simulink library "dyn_lib"  (R2023b)
settings: Solver=VariableStepAuto  StartTime=0.0  StopTime=10.0  RelTol=1e-3
undefined symbols (not defined in the file or in its folder): earth_radius, sun_radius, v0, x0
libraries: $bdroot x5, vrlib x3, matrix_library x1
settings Model: Creator=brent  LastModifiedBy=brent

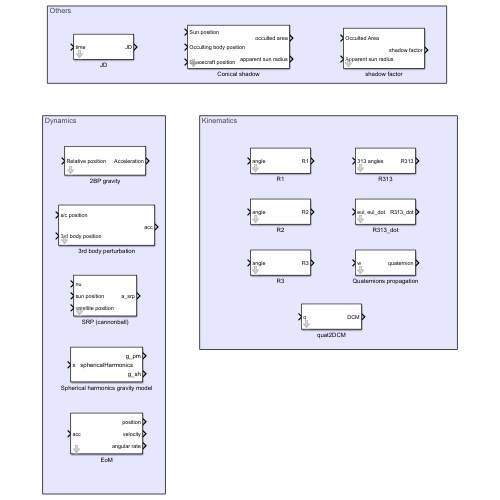
[thumbnail: Simulink's stored preview of the top-level diagram]
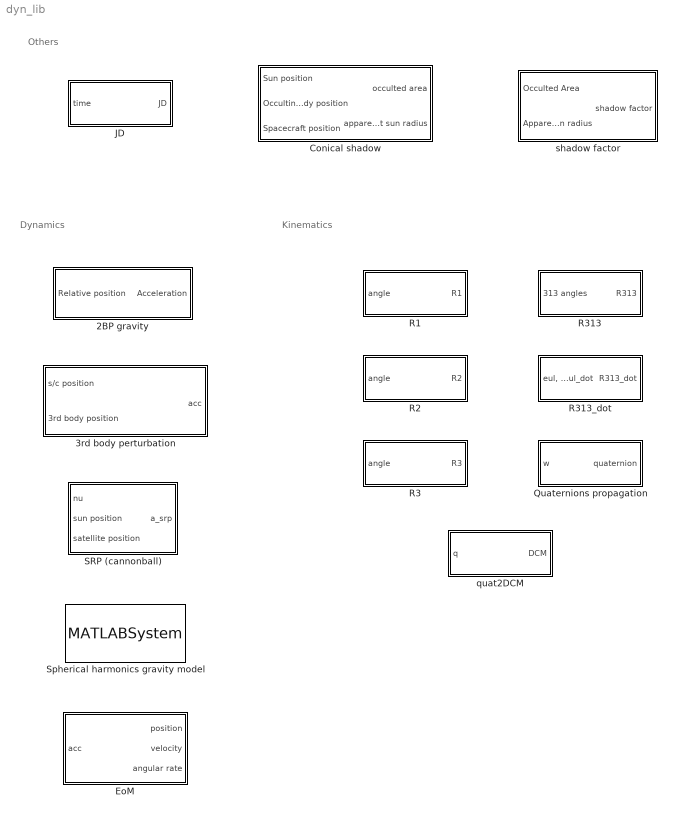
== system dyn_lib ==
  note: Kinematics
  note: Others
  note: Dynamics
  2BP gravity : Subsystem  mask{mu=0}
      mask prompts: mu "Celestial body's gravitational constant"
      mask DialogControl DescGroupVar Prompt: 2BP gravity
      mask DialogControl DescTextVar Prompt: Gravitational acceleration caused by one point mass, according to the two-body problem theory
  3rd body perturbation : Subsystem  mask{mu=sqrt(3)^3}
      mask prompts: mu "3rd body mu"
      mask DialogControl DescGroupVar Prompt: 3rd body perturbation
  Conical shadow : Subsystem  mask{R_B=earth_radius, R_S=sun_radius}
      mask prompts: R_B "Occulting body radius"; R_S "Sun Radius"
  EoM : Subsystem  mask{x0=x0, v0=v0}
      mask prompts: x0 "Initial position"; v0 "Initial velocity"
      mask DialogControl DescGroupVar Prompt: Equations of motion
  JD : Subsystem  mask{year=0, month=0, day=0, hour=0, min=0, sec=0}
      mask prompts: min "Minutes"; sec "Seconds"
      mask DialogControl DescGroupVar Prompt: Julian Date
      mask DialogControl DescTextVar Prompt: Compute the julian date computed as the sum of the parameter date and input seconds
      mask DialogControl ParameterGroupVar Prompt: Date
  Quaternions propagation : Subsystem  mask{q0=0}
      mask prompts: q0 "Initial attitude quaternion"
      mask DialogControl DescGroupVar Prompt: Quaternion propagation
  R1 : Subsystem
      mask DialogControl DescGroupVar Prompt: R1
      mask DialogControl DescTextVar Prompt: Rotate the reference frame of an angle alpha around the x axis. To rotate a vector and keep constant the reference frame, premultiply the vector by the transpose of this matrix
  R2 : Subsystem
      mask DialogControl DescGroupVar Prompt: R2
      mask DialogControl DescTextVar Prompt: Rotate the reference frame of an angle alpha around the y axis. To rotate a vector and keep constant the reference frame, premultiply the vector by the transpose of this matrix
  R3 : Subsystem
      mask DialogControl DescGroupVar Prompt: R3
      mask DialogControl DescTextVar Prompt: Rotate the reference frame of an angle alpha around the z axis. To rotate a vector and keep constant the reference frame, premultiply the vector by the transpose of this matrix.
  R313 : Subsystem
      mask DialogControl DescGroupVar Prompt: R313
      mask DialogControl DescTextVar Prompt: Rotate the reference frame with a 313 rotation series around the y axis. To rotate a vector and keep constant the reference frame, premultiply the vector by the transpose of this matrix
  R313_dot : Subsystem
      mask DialogControl DescGroupVar Prompt: R313_dot
      mask DialogControl DescTextVar Prompt: Time derivative of the 313 roation matrix
  SRP (cannonball) : Subsystem  mask{C_R=0, A_sc=0, m=0, AU=0, P=0}
      mask prompts: C_R "Radiation pressure coefficient"; A_sc "Spacecraft area"; m "Spacecraft mass"; AU "Astronomical units conversion"; P "Radiation pressure"
      mask DialogControl DescGroupVar Prompt: Solar Radiation Pressure
  Spherical harmonics gravity model : MATLABSystem  System=sphericalHarmonics  body_coeffs=[]  mu=[]  ref_radius=[]  nMax=[]  mMax=[]  SimulateUsing=Code generation
      mask Type: sphericalHarmonics
      mask Display:
      | disp('sphericalHarmonics');
      | port_label('input',1,'x');
      | port_label('output',1,'g_pm');
      | port_label('output',2,'g_sh');
  quat2DCM : Subsystem
      mask DialogControl DescGroupVar Prompt: quat2DCM
      mask DialogControl DescTextVar Prompt: convert a quaternion (scalar last) into the corresponding  rotation matrix
  shadow factor : Subsystem
      mask DialogControl DescGroupVar Prompt: Shadow factor

== system dyn_lib/2BP gravity ==
  note: $a = -\mu\frac{r}{|r|^3}$
  note: Two body problem equation
      |
      | Source:
      | H. D. Curtis, Orbital Mechanics for Engineering Students
  Relative position : Inport
  Constant : Constant  Value=3
  Constant1 : Constant  Value=mu
  Divide : Product  Inputs=*/
  Dot Product : DotProduct  OutDataTypeStr=Inherit: Inherit via internal rule
  Gain : Gain  Gain=-1
  Power : Math  Operator=pow
  Product : Product
  Square Root : Sqrt
  Acceleration : Outport
  wires:
  Square Root/1 -> Power/1
  Constant/1 -> Power/2
  Constant1/1 -> Divide/1
  Power/1 -> Divide/2
  Divide/1 -> Product/2
  Product/1 -> Gain/1
  Relative position/1 -> Dot Product/2, Dot Product/1, Product/1
  Dot Product/1 -> Square Root/1
  Gain/1 -> Acceleration/1

== system dyn_lib/3rd body perturbation ==
  note: $a = -\mu_3\frac{r_s - r_3}{|r_s - r_3|^3}$
  note: Gravitational perturbation due to the presence of a third body
      |
      | Source:
      | H. D. Curtis, Orbital Mechanics for Engineering Students
  s/c position : Inport
  3rd body position : Inport  Port=2
  2BP gravity : $bdroot/2BP gravity  mu=mu
  2BP gravity10 : $bdroot/2BP gravity  mu=mu
  Add2 : Sum  Inputs=+-
  Subtract : Sum
  acc : Outport
  wires:
  Add2/1 -> 2BP gravity/1
  s/c position/1 -> Add2/1  "satellite postion"
  2BP gravity/1 -> Subtract/1
  2BP gravity10/1 -> Subtract/2
  3rd body position/1 -> 2BP gravity10/1, Add2/2  "3rd body position"
  Subtract/1 -> acc/1  "acc"

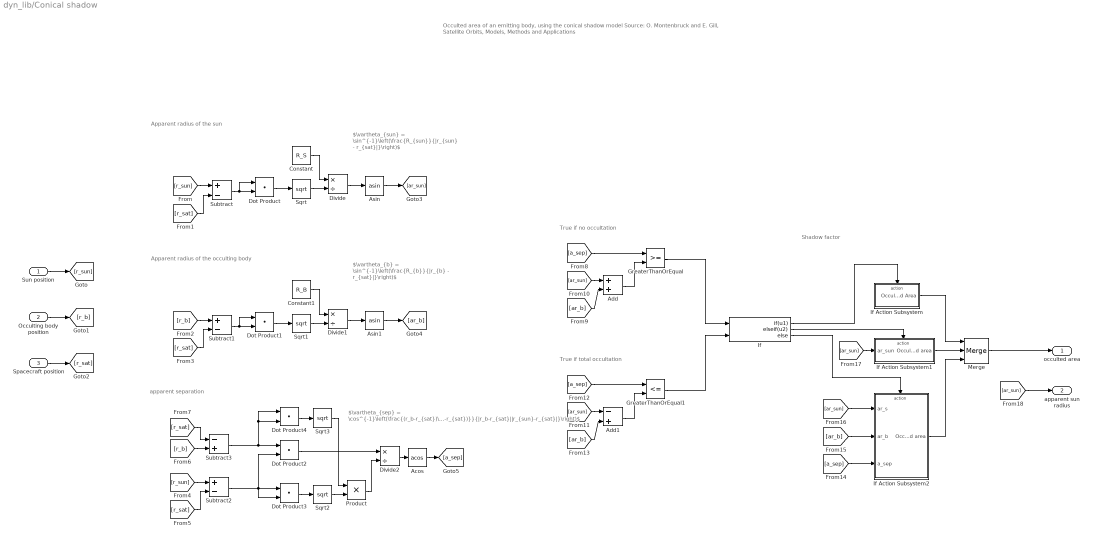
== system dyn_lib/Conical shadow ==
  note: $\vartheta_{b} = \sin^{-1}\left(\frac{R_{b}}{|r_{b} - r_{sat}|}\right)$
  note: Occulted area of an emitting body, using the conical shadow model
      |
      | Source:
      | O. Montenbruck and E. Gill, Satellite Orbits, Models, Methods and Applications
  note: Shadow factor
  note: True if no occultation
  note: apparent separation
  note: Apparent radius of the sun
  note: Apparent radius of the occulting body
  note: True if total occultation
  note: $\vartheta_{sun} = \sin^{-1}\left(\frac{R_{sun}}{|r_{sun} - r_{sat}|}\right)$
  note: $\vartheta_{sep} = \cos^{-1}\left(\frac{(r_b-r_{sat})\cdot{(r_{sun}-r_{sat})}}{|r_b-r_{sat}||r_{sun}-r_{sat}|}\right)$
  Sun position : Inport
  Occulting body position : Inport  Port=2
  Spacecraft position : Inport  Port=3
  Acos : Trigonometry  Operator=acos
  Add : Sum
  Add1 : Sum  Inputs=-+
  Asin : Trigonometry  Operator=asin
  Asin1 : Trigonometry  Operator=asin
  Constant : Constant  Value=R_S
  Constant1 : Constant  Value=R_B
  Divide : Product  Inputs=*/
  Divide1 : Product  Inputs=*/
  Divide2 : Product  Inputs=*/
  Dot Product{,1..4} (5 alike) : DotProduct  OutDataTypeStr=Inherit: Inherit via internal rule
  GreaterThanOrEqual : RelationalOperator  OutDataTypeStr=boolean  RndMeth=Simplest  InputSameDT=off
  GreaterThanOrEqual1 : RelationalOperator  Operator=<=  OutDataTypeStr=boolean  RndMeth=Simplest  InputSameDT=off
  If : If  NumInputs=2  IfExpression=u1  ElseIfExpressions=u2
  If Action Subsystem : Subsystem  TreatAsAtomicUnit=on
  If Action Subsystem1 : Subsystem  TreatAsAtomicUnit=on
  If Action Subsystem2 : Subsystem  TreatAsAtomicUnit=on
  Merge : Merge  Inputs=3
  Product : Product
  Sqrt{,1..3} (4 alike) : Sqrt
  Subtract : Sum  Inputs=+-
  Subtract1 : Sum  Inputs=+-
  Subtract2 : Sum  Inputs=+-
  Subtract3 : Sum  Inputs=-+
  occulted area : Outport
  apparent sun radius : Outport  Port=2
  wires:
  Divide2/1 -> Acos/1
  Acos/1 -> [a_sep]
  Sun position/1 -> [r_sun]
  Occulting body position/1 -> [r_b]
  Spacecraft position/1 -> [r_sat]
  [r_sun] -> Subtract/1
  [r_sat] -> Subtract/2
  Subtract/1 -> Dot Product/1, Dot Product/2
  Dot Product/1 -> Sqrt/1
  Constant/1 -> Divide/1
  Sqrt/1 -> Divide/2
  Divide/1 -> Asin/1
  Asin/1 -> [ar_sun]
  Asin1/1 -> [ar_b]
  Divide1/1 -> Asin1/1
  Sqrt1/1 -> Divide1/2
  Constant1/1 -> Divide1/1
  [r_b] -> Subtract1/1
  Dot Product1/1 -> Sqrt1/1
  Subtract1/1 -> Dot Product1/1, Dot Product1/2
  [r_sat] -> Subtract1/2
  [r_sun] -> Subtract2/1
  [r_sat] -> Subtract2/2
  [r_b] -> Subtract3/2
  [r_sat] -> Subtract3/1
  Subtract3/1 -> Dot Product4/2, Dot Product4/1, Dot Product2/1
  Subtract2/1 -> Dot Product3/2, Dot Product3/1, Dot Product2/2
  Dot Product2/1 -> Divide2/1
  Dot Product3/1 -> Sqrt2/1
  Dot Product4/1 -> Sqrt3/1
  Sqrt2/1 -> Product/2
  Sqrt3/1 -> Product/1
  Product/1 -> Divide2/2
  [a_sep] -> GreaterThanOrEqual/1
  [ar_sun] -> Add/1
  [ar_b] -> Add/2
  Add/1 -> GreaterThanOrEqual/2
  GreaterThanOrEqual/1 -> If/1
  If/1 -> If Action Subsystem/Action
  Add1/1 -> GreaterThanOrEqual1/2
  [a_sep] -> GreaterThanOrEqual1/1
  [ar_b] -> Add1/2
  GreaterThanOrEqual1/1 -> If/2
  [ar_sun] -> Add1/1
  If/2 -> If Action Subsystem1/Action
  If/3 -> If Action Subsystem2/Action
  [a_sep] -> If Action Subsystem2/3(a_sep)
  [ar_b] -> If Action Subsystem2/2(ar_b)
  [ar_sun] -> If Action Subsystem2/1(ar_s)
  If Action Subsystem1/1(Occulted area) -> Merge/2
  If Action Subsystem/1(Occulted Area) -> Merge/1
  If Action Subsystem2/1(Occulted area) -> Merge/3
  Merge/1 -> occulted area/1
  [ar_sun] -> If Action Subsystem1/1(ar_sun)
  [ar_sun] -> apparent sun radius/1

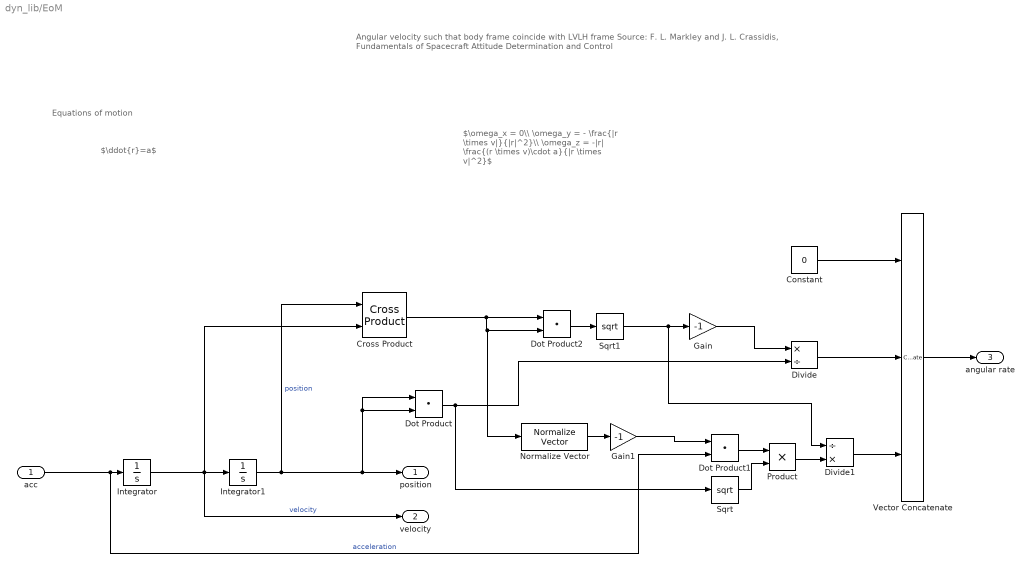
== system dyn_lib/EoM ==
  note: $\omega_x = 0\\ \omega_y = - \frac{|r \times v|}{|r|^2}\\ \omega_z = -|r| \frac{(r \times v)\cdot a}{|r \times v|^2}$
  note: Angular velocity such that body frame coincide with LVLH frame
      |
      | Source:
      | F. L. Markley and J. L. Crassidis, Fundamentals of Spacecraft Attitude Determination
      | and Control
  note: $\ddot{r}=a$
  note: Equations of motion
  acc : Inport
  Constant : Constant  Value=0
  Cross Product : matrix_library/Cross Product
  Divide : Product  Inputs=*/
  Divide1 : Product  Inputs=/*
  Dot Product : DotProduct  OutDataTypeStr=Inherit: Inherit via internal rule
  Dot Product1 : DotProduct  OutDataTypeStr=Inherit: Inherit via internal rule
  Dot Product2 : DotProduct  OutDataTypeStr=Inherit: Inherit via internal rule
  Gain : Gain  Gain=-1
  Gain1 : Gain  Gain=-1
  Integrator : Integrator  InitialCondition=v0
  Integrator1 : Integrator  InitialCondition=x0
  Normalize Vector : vrlib/Utilities/Normalize Vector  maxzero=0
  Product : Product
  Sqrt : Sqrt
  Sqrt1 : Sqrt
  Vector Concatenate : Concatenate  NumInputs=3
  position : Outport
  velocity : Outport  Port=2
  angular rate : Outport  Port=3
  wires:
  Normalize Vector/1 -> Gain1/1
  Gain/1 -> Divide/1
  Constant/1 -> Vector Concatenate/1
  Divide/1 -> Vector Concatenate/2
  Divide1/1 -> Vector Concatenate/3
  Sqrt1/1 -> Divide1/1, Gain/1
  Dot Product2/1 -> Sqrt1/1
  Product/1 -> Divide1/2
  Sqrt/1 -> Product/2
  Dot Product1/1 -> Product/1
  Gain1/1 -> Dot Product1/1
  Cross Product/1 -> Dot Product2/2, Normalize Vector/1, Dot Product2/1
  Dot Product/1 -> Sqrt/1, Divide/2
  Integrator/1 -> Cross Product/2, velocity/1, Integrator1/1  "velocity"
  acc/1 -> Dot Product1/2, Integrator/1  "acceleration"
  Integrator1/1 -> Cross Product/1, position/1, Dot Product/2, Dot Product/1  "position"
  Vector Concatenate/1 -> angular rate/1

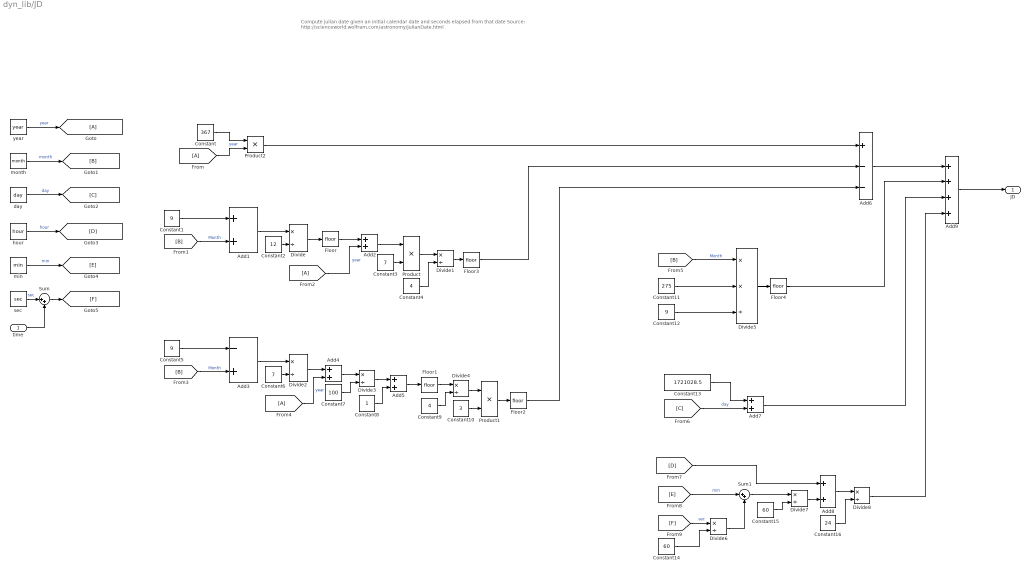
== system dyn_lib/JD ==
  note: Compute julian date given an initial calendar date and seconds elapsed from that date
      |
      | Source:
      | http://scienceworld.wolfram.com/astronomy/JulianDate.html
  time : Inport
  Add{1..2,4..5,7..8} (6 alike) : Sum
  Add3 : Sum  Inputs=-+
  Add6 : Sum  Inputs=+--
  Add9 : Sum  Inputs=++++
  Constant : Constant  Value=367
  Constant1 : Constant  Value=9
  Constant10 : Constant  Value=3
  Constant11 : Constant  Value=275
  Constant12 : Constant  Value=9
  Constant13 : Constant  Value=1721028.5
  Constant14 : Constant  Value=60
  Constant15 : Constant  Value=60
  Constant16 : Constant  Value=24
  Constant2 : Constant  Value=12
  Constant3 : Constant  Value=7
  Constant4 : Constant  Value=4
  Constant5 : Constant  Value=9
  Constant6 : Constant  Value=7
  Constant7 : Constant  Value=100
  Constant8 : Constant
  Constant9 : Constant  Value=4
  Divide{,1..4,6..8} (8 alike) : Product  Inputs=*/
  Divide5 : Product  Inputs=**/
  Floor{,1..4} (5 alike) : Rounding
  From : From
  From2 : From
  From4 : From
  Goto : Goto
  Product : Product
  Product1 : Product
  Product2 : Product
  Sum : Sum  Inputs=|++
  Sum1 : Sum  Inputs=|++
  day : Constant  Value=day
  hour : Constant  Value=hour
  min : Constant  Value=min
  month : Constant  Value=month
  sec : Constant  Value=sec
  year : Constant  Value=year
  JD : Outport
  wires:
  year/1 -> Goto/1  "year"
  month/1 -> [B]  "month"
  day/1 -> [C]  "day"
  Constant/1 -> Product2/1
  From/1 -> Product2/2  "year"
  [B] -> Add1/2  "Month"
  Constant1/1 -> Add1/1
  Add1/1 -> Divide/1
  Constant2/1 -> Divide/2
  Divide/1 -> Floor/1
  From2/1 -> Add2/2  "year"
  Floor/1 -> Add2/1
  Add2/1 -> Product/1
  Constant3/1 -> Product/2
  Product/1 -> Divide1/1
  Constant4/1 -> Divide1/2
  From4/1 -> Add4/2  "year"
  Add3/1 -> Divide2/1
  Constant7/1 -> Divide3/2
  Constant6/1 -> Divide2/2
  [B] -> Add3/2  "Month"
  Add4/1 -> Divide3/1
  Divide2/1 -> Add4/1
  Constant5/1 -> Add3/1
  Divide3/1 -> Add5/1
  Constant8/1 -> Add5/2
  Add5/1 -> Floor1/1
  Floor1/1 -> Divide4/1
  Constant9/1 -> Divide4/2
  Divide4/1 -> Product1/1
  Constant10/1 -> Product1/2
  Product1/1 -> Floor2/1
  Divide1/1 -> Floor3/1
  Product2/1 -> Add6/1
  Floor3/1 -> Add6/2
  Floor2/1 -> Add6/3
  [B] -> Divide5/1  "Month"
  Constant11/1 -> Divide5/2
  Constant12/1 -> Divide5/3
  [C] -> Add7/2  "day"
  Constant13/1 -> Add7/1
  min/1 -> [E]  "min"
  hour/1 -> [D]  "hour"
  sec/1 -> Sum/1  "sec"
  time/1 -> Sum/2
  Sum/1 -> [F]
  Constant14/1 -> Divide6/2
  [F] -> Divide6/1  "sec"
  Divide6/1 -> Sum1/2
  [E] -> Sum1/1  "min"
  Sum1/1 -> Divide7/1
  Constant15/1 -> Divide7/2
  Divide7/1 -> Add8/2
  [D] -> Add8/1
  Constant16/1 -> Divide8/2
  Add8/1 -> Divide8/1
  Add6/1 -> Add9/1
  Divide5/1 -> Floor4/1
  Add7/1 -> Add9/3
  Divide8/1 -> Add9/4
  Add9/1 -> JD/1
  Floor4/1 -> Add9/2

== system dyn_lib/Quaternions propagation ==
  note: $\dot{q} = \frac{1}{2}\Omega q$
  note: Quaternion propagation
      |
      | Source:
      | J. R. Wertz, Spacecraft Attitude Determination and Control
  w : Inport
  Create matrix OMEGA : Subsystem
  Gain : Gain  Gain=1/2  SaturateOnIntegerOverflow=on  OutDataTypeStr=Inherit: Same as input  ParamDataTypeStr=Inherit: Same as input
  Integrator2 : Integrator  InitialCondition=q0
  Matrix Multiply : Product  Multiplication=Matrix(*)
  Normalize Vector : vrlib/Utilities/Normalize Vector  maxzero=0
  quaternion : Outport
  wires:
  w/1 -> Create matrix OMEGA/1(w)
  Matrix Multiply/1 -> Integrator2/1  "q_dot"
  Normalize Vector/1 -> quaternion/1, Matrix Multiply/2  "q_norm"
  Integrator2/1 -> Normalize Vector/1  "q"
  Create matrix OMEGA/1(OMEGA) -> Gain/1
  Gain/1 -> Matrix Multiply/1

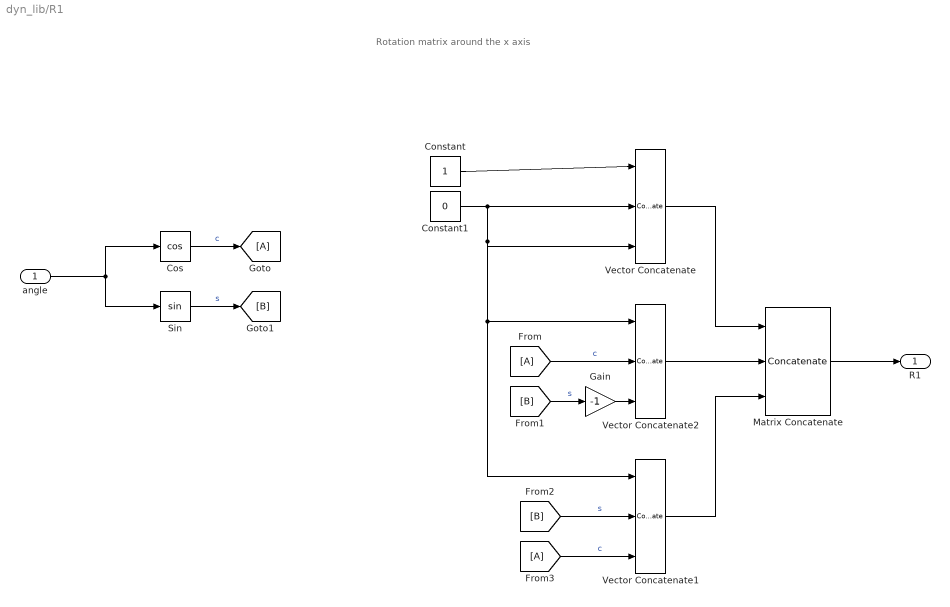
== system dyn_lib/R1 ==
  note: Rotation matrix around the x axis
  angle : Inport
  Constant : Constant
  Constant1 : Constant  Value=0
  Cos : Trigonometry  Operator=cos
  From : From
  From3 : From
  Gain : Gain  Gain=-1
  Goto : Goto
  Matrix Concatenate : Concatenate  NumInputs=3  Mode=Multidimensional array  ConcatenateDimension=2
  Sin : Trigonometry
  Vector Concatenate : Concatenate  NumInputs=3
  Vector Concatenate1 : Concatenate  NumInputs=3
  Vector Concatenate2 : Concatenate  NumInputs=3
  R1 : Outport
  wires:
  angle/1 -> Cos/1, Sin/1
  Cos/1 -> Goto/1  "c"
  Sin/1 -> [B]  "s"
  Constant/1 -> Vector Concatenate/1
  Constant1/1 -> Vector Concatenate/2, Vector Concatenate/3, Vector Concatenate1/1, Vector Concatenate2/1
  From/1 -> Vector Concatenate2/2  "c"
  [B] -> Gain/1  "s"
  Gain/1 -> Vector Concatenate2/3
  [B] -> Vector Concatenate1/2  "s"
  From3/1 -> Vector Concatenate1/3  "c"
  Vector Concatenate2/1 -> Matrix Concatenate/2
  Vector Concatenate1/1 -> Matrix Concatenate/3
  Vector Concatenate/1 -> Matrix Concatenate/1
  Matrix Concatenate/1 -> R1/1

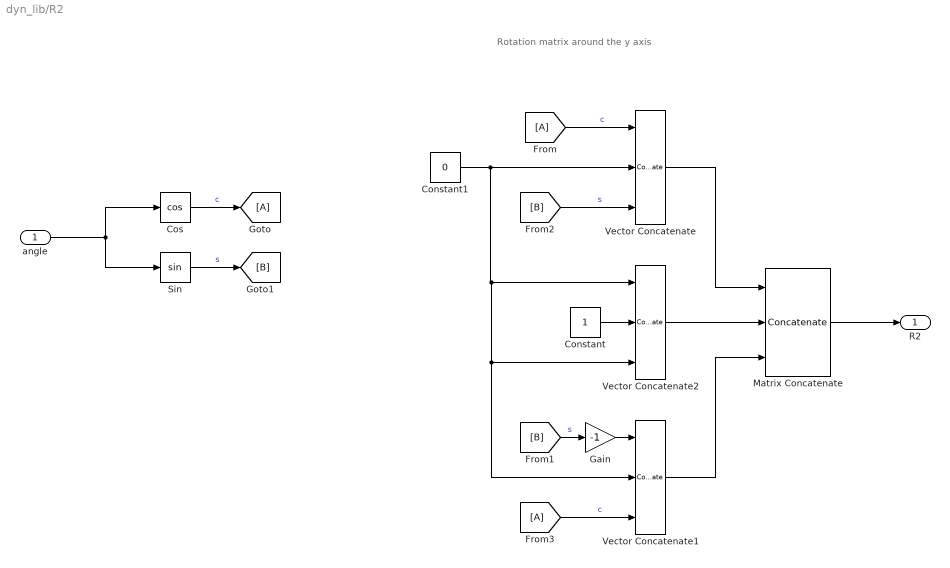
== system dyn_lib/R2 ==
  note: Rotation matrix around the y axis
  angle : Inport
  Constant : Constant
  Constant1 : Constant  Value=0
  Cos : Trigonometry  Operator=cos
  From : From
  From3 : From
  Gain : Gain  Gain=-1
  Goto : Goto
  Matrix Concatenate : Concatenate  NumInputs=3  Mode=Multidimensional array  ConcatenateDimension=2
  Sin : Trigonometry
  Vector Concatenate : Concatenate  NumInputs=3
  Vector Concatenate1 : Concatenate  NumInputs=3
  Vector Concatenate2 : Concatenate  NumInputs=3
  R2 : Outport
  wires:
  Matrix Concatenate/1 -> R2/1
  Vector Concatenate2/1 -> Matrix Concatenate/2
  Vector Concatenate/1 -> Matrix Concatenate/1
  Vector Concatenate1/1 -> Matrix Concatenate/3
  [B] -> Gain/1  "s"
  Cos/1 -> Goto/1  "c"
  Sin/1 -> [B]  "s"
  angle/1 -> Cos/1, Sin/1
  From/1 -> Vector Concatenate/1  "c"
  Constant1/1 -> Vector Concatenate1/2, Vector Concatenate2/3, Vector Concatenate2/1, Vector Concatenate/2
  [B] -> Vector Concatenate/3  "s"
  Constant/1 -> Vector Concatenate2/2
  Gain/1 -> Vector Concatenate1/1
  From3/1 -> Vector Concatenate1/3  "c"

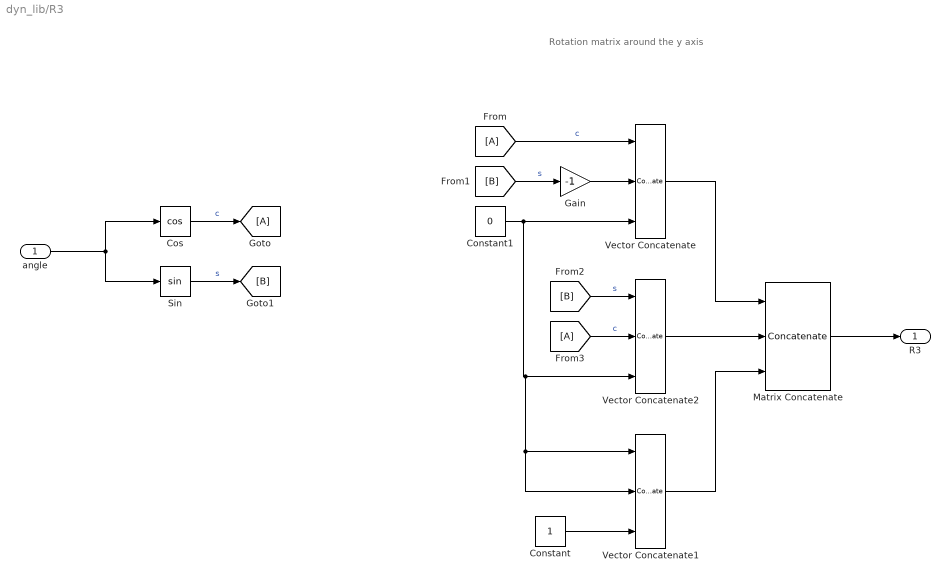
== system dyn_lib/R3 ==
  note: Rotation matrix around the y axis
  angle : Inport
  Constant : Constant
  Constant1 : Constant  Value=0
  Cos : Trigonometry  Operator=cos
  From : From
  From3 : From
  Gain : Gain  Gain=-1
  Goto : Goto
  Matrix Concatenate : Concatenate  NumInputs=3  Mode=Multidimensional array  ConcatenateDimension=2
  Sin : Trigonometry
  Vector Concatenate : Concatenate  NumInputs=3
  Vector Concatenate1 : Concatenate  NumInputs=3
  Vector Concatenate2 : Concatenate  NumInputs=3
  R3 : Outport
  wires:
  Cos/1 -> Goto/1  "c"
  angle/1 -> Cos/1, Sin/1
  Sin/1 -> [B]  "s"
  Vector Concatenate2/1 -> Matrix Concatenate/2
  Vector Concatenate1/1 -> Matrix Concatenate/3
  [B] -> Gain/1  "s"
  Vector Concatenate/1 -> Matrix Concatenate/1
  Matrix Concatenate/1 -> R3/1
  From/1 -> Vector Concatenate/1  "c"
  Gain/1 -> Vector Concatenate/2
  Constant1/1 -> Vector Concatenate1/1, Vector Concatenate1/2, Vector Concatenate2/3, Vector Concatenate/3
  [B] -> Vector Concatenate2/1  "s"
  From3/1 -> Vector Concatenate2/2  "c"
  Constant/1 -> Vector Concatenate1/3

== system dyn_lib/R313 ==
  note: Rotation matrix for the ZXZ sequence of rotations
  313 angles : Inport
  Demux : Demux  Outputs=3
  Matrix Multiply : Product  Inputs=3  Multiplication=Matrix(*)
  R1 : $bdroot/R1
  R3_1 : $bdroot/R3
  R3_2 : $bdroot/R3
  R313 : Outport
  wires:
  313 angles/1 -> Demux/1
  Demux/1 -> R3_1/1
  Demux/2 -> R1/1
  Demux/3 -> R3_2/1
  Matrix Multiply/1 -> R313/1
  R1/1 -> Matrix Multiply/2
  R3_1/1 -> Matrix Multiply/1
  R3_2/1 -> Matrix Multiply/3

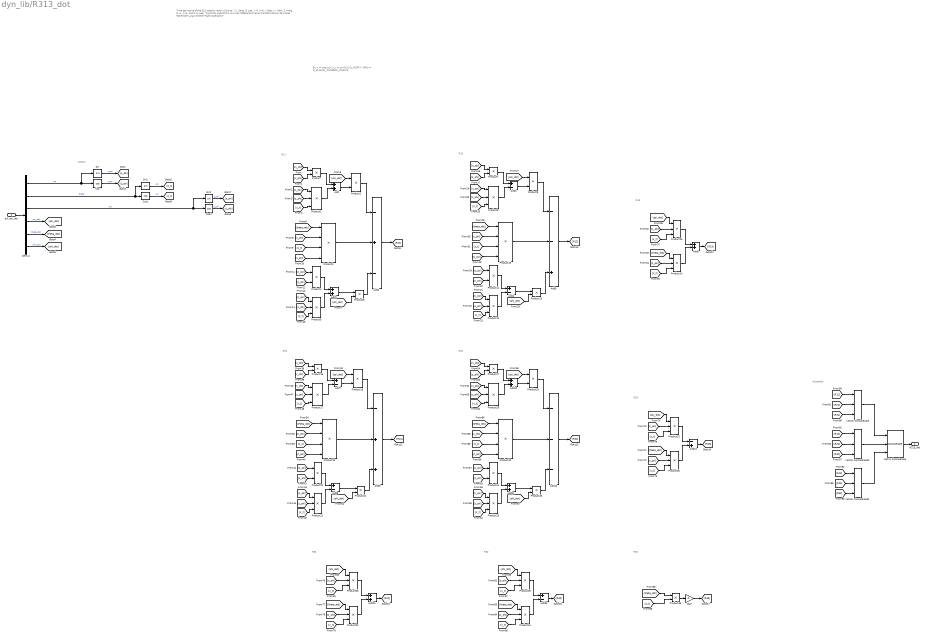
== system dyn_lib/R313_dot ==
  note: $c_x = \cos{x}\\ s_x = \sin{x}\\ D_{ICRF}^{PA} = R_3(\psi)R_1(\theta)R_3(\phi)$
  note: Time derivative of the 313 rotation matrix
      |
      | Source:
      | Y.-J. Song, D. Lee, Y.-R. Kim, J. Bae, J.-i. Park, S. Hong, D.-K. Kim, and S.-R. Lee, “Practical Algorithms on Lunar Reference Frame Transformations for Korea Pathfinder Lunar Orbiter Flight Operation”
  note: Assembly
  note: R13
  note: R11
  note: cos/sin
  note: R12
  note: R21
  note: R22
  note: R23
  note: R31
  note: R32
  note: R33
  "eul, eul_dot" : Inport
  Add{,1,6,10..11,14} (6 alike) : Sum
  Add12 : Sum  Inputs=---
  Add13 : Sum  Inputs=-+
  Add{3..4,7..8,15} (5 alike) : Sum  Inputs=+-
  Add2 : Sum  Inputs=-+-
  Add5 : Sum  Inputs=--+
  Add9 : Sum  Inputs=-++
  Cos : Trigonometry  Operator=cos
  Cos1 : Trigonometry  Operator=cos
  Cos2 : Trigonometry  Operator=cos
  Demux : Demux  Outputs=6
  Gain : Gain  Gain=-1
  Matrix Concatenate : Concatenate  NumInputs=3  Mode=Multidimensional array  ConcatenateDimension=2
  Product{,2,4,6..7,9,11,13,16,18,20,22,24,26..27,29,36} (17 alike) : Product
  Product{1,5,8,12,14..15,17,21,25,28,30..35} (16 alike) : Product  Inputs=3
  Product{3,10,19,23} (4 alike) : Product  Inputs=4
  Sin : Trigonometry
  Sin1 : Trigonometry
  Sin2 : Trigonometry
  Vector Concatenate : Concatenate  NumInputs=3
  Vector Concatenate1 : Concatenate  NumInputs=3
  Vector Concatenate2 : Concatenate  NumInputs=3
  R313_dot : Outport
  wires:
  "eul, eul_dot"/1 -> Demux/1
  Demux/1 -> Sin/1, Cos/1  "psi"
  Demux/4 -> [psi_dot]  "psi_dot"
  Demux/5 -> [theta_dot]  "theta_dot"
  Demux/6 -> [phi_dot]  "phi_dot"
  Demux/2 -> Sin1/1, Cos1/1  "theta"
  Demux/3 -> Cos2/1, Sin2/1  "phi"
  Sin/1 -> [s_psi]  "s_psi"
  Cos/1 -> [c_psi]  "c_psi"
  Sin1/1 -> [s_t]  "s_t"
  Cos1/1 -> [c_t]  "c_t"
  Sin2/1 -> [s_phi]  "s_phi"
  Cos2/1 -> [c_phi]  "c_phi"
  [s_psi] -> Product/1
  [c_phi] -> Product/2
  [s_phi] -> Product1/2
  [c_psi] -> Product1/1
  [c_t] -> Product1/3
  Product1/1 -> Add/2
  Product/1 -> Add/1
  Add/1 -> Product2/2
  [psi_dot] -> Product2/1
  [s_phi] -> Product3/2
  [s_t] -> Product3/3
  [theta_dot] -> Product3/1
  [s_psi] -> Product3/4
  [c_psi] -> Product4/1
  [s_phi] -> Product4/2
  [c_phi] -> Product5/2
  [c_t] -> Product5/3
  [s_psi] -> Product5/1
  Product5/1 -> Add1/2
  Product4/1 -> Add1/1
  Add1/1 -> Product6/1
  [phi_dot] -> Product6/2
  Product6/1 -> Add2/3
  Product3/1 -> Add2/2
  Product2/1 -> Add2/1
  Add2/1 -> [R11]
  [c_t] -> Product12/3
  [s_psi] -> Product10/4
  Product10/1 -> Add5/2
  [c_psi] -> Product11/1
  [theta_dot] -> Product10/1
  [c_phi] -> Product8/2
  Product9/1 -> Add5/1
  Product13/1 -> Add5/3
  [s_psi] -> Product12/1
  [s_psi] -> Product7/1
  [phi_dot] -> Product13/2
  [c_phi] -> Product10/2
  Add3/1 -> Product9/2
  [psi_dot] -> Product9/1
  [c_phi] -> Product11/2
  Product11/1 -> Add4/1
  [s_phi] -> Product7/2
  Product12/1 -> Add4/2
  [c_psi] -> Product8/1
  Product7/1 -> Add3/1
  Add4/1 -> Product13/1
  Product8/1 -> Add3/2
  [c_t] -> Product8/3
  Add5/1 -> [R12]
  [s_phi] -> Product12/2
  [s_t] -> Product10/3
  [s_psi] -> Product14/2
  [theta_dot] -> Product14/1
  [c_t] -> Product14/3
  [c_psi] -> Product15/2
  [psi_dot] -> Product15/1
  [s_t] -> Product15/3
  Product15/1 -> Add6/1
  Product14/1 -> Add6/2
  Add6/1 -> [R13]
  Add9/1 -> [R21]
  Product18/1 -> Add9/1
  Product19/1 -> Add9/2
  Product22/1 -> Add9/3
  [phi_dot] -> Product22/2
  Add8/1 -> Product22/1
  Product20/1 -> Add8/1
  Product21/1 -> Add8/2
  [c_psi] -> Product21/1
  [c_t] -> Product21/3
  [c_phi] -> Product21/2
  [s_phi] -> Product20/2
  [s_psi] -> Product20/1
  [c_psi] -> Product19/4
  [theta_dot] -> Product19/1
  [s_t] -> Product19/3
  [s_phi] -> Product19/2
  [psi_dot] -> Product18/1
  Add7/1 -> Product18/2
  Product16/1 -> Add7/1
  Product17/1 -> Add7/2
  [c_t] -> Product17/3
  [s_phi] -> Product17/1
  [s_psi] -> Product17/2
  [c_phi] -> Product16/2
  [c_psi] -> Product16/1
  Add11/1 -> Product26/1
  [s_phi] -> Product25/2
  [s_psi] -> Product28/1
  Product28/1 -> Add10/2
  Product27/1 -> Add10/1
  Product25/1 -> Add11/2
  Add12/1 -> [R22]
  [c_t] -> Product28/3
  [s_phi] -> Product27/2
  [c_psi] -> Product25/1
  [psi_dot] -> Product29/1
  Add10/1 -> Product29/2
  Product26/1 -> Add12/3
  [c_phi] -> Product24/2
  [c_psi] -> Product27/1
  Product24/1 -> Add11/1
  [c_phi] -> Product28/2
  Product29/1 -> Add12/1
  [phi_dot] -> Product26/2
  [s_psi] -> Product24/1
  [c_psi] -> Product23/4
  [s_t] -> Product23/3
  [theta_dot] -> Product23/1
  [c_t] -> Product25/3
  [c_phi] -> Product23/2
  Product23/1 -> Add12/2
  [c_t] -> Product30/3
  [psi_dot] -> Product31/1
  Product30/1 -> Add13/2
  [c_psi] -> Product30/2
  Product31/1 -> Add13/1
  [theta_dot] -> Product30/1
  Add13/1 -> [R23]
  [s_psi] -> Product31/2
  [s_t] -> Product31/3
  [theta_dot] -> Product32/1
  [s_t] -> Product33/3
  [c_phi] -> Product33/2
  [phi_dot] -> Product33/1
  [c_t] -> Product32/3
  Product33/1 -> Add14/1
  [s_phi] -> Product32/2
  Add14/1 -> [R31]
  Product32/1 -> Add14/2
  Product34/1 -> Add15/2
  [s_t] -> Product35/3
  [theta_dot] -> Product34/1
  [c_t] -> Product34/3
  [s_phi] -> Product35/2
  [phi_dot] -> Product35/1
  Add15/1 -> [R32]
  Product35/1 -> Add15/1
  [c_phi] -> Product34/2
  [theta_dot] -> Product36/1
  [s_t] -> Product36/2
  Product36/1 -> Gain/1
  Gain/1 -> [R33]
  Vector Concatenate2/1 -> Matrix Concatenate/2
  Vector Concatenate/1 -> Matrix Concatenate/1
  Vector Concatenate1/1 -> Matrix Concatenate/3
  [R11] -> Vector Concatenate/1
  [R21] -> Vector Concatenate/2
  [R31] -> Vector Concatenate/3
  [R22] -> Vector Concatenate2/2
  [R12] -> Vector Concatenate2/1
  [R32] -> Vector Concatenate2/3
  [R13] -> Vector Concatenate1/1
  [R23] -> Vector Concatenate1/2
  [R33] -> Vector Concatenate1/3
  Matrix Concatenate/1 -> R313_dot/1

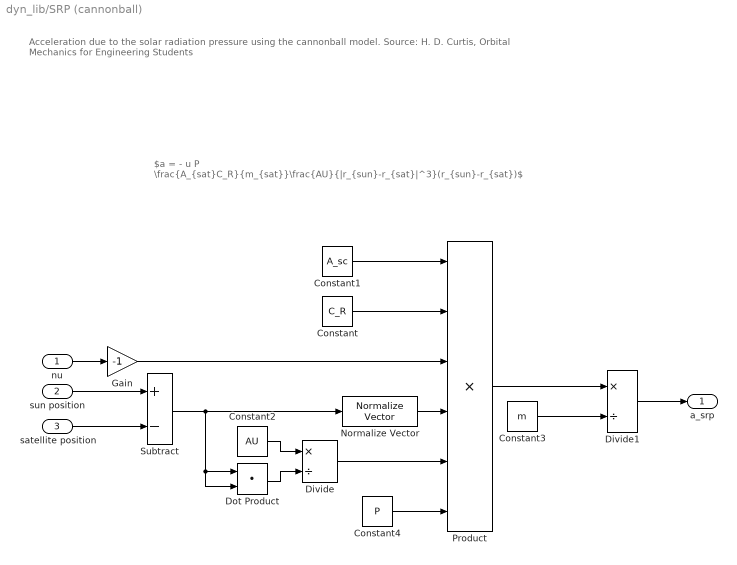
== system dyn_lib/SRP (cannonball) ==
  note: Acceleration due to the solar radiation pressure using the cannonball model.
      |
      | Source:
      | H. D. Curtis, Orbital Mechanics for Engineering Students
  note: $a = -\nu P \frac{A_{sat}C_R}{m_{sat}}\frac{AU}{|r_{sun}-r_{sat}|^3}(r_{sun}-r_{sat})$
  nu : Inport
  sun position : Inport  Port=2
  satellite position : Inport  Port=3
  Constant : Constant  Value=C_R
  Constant1 : Constant  Value=A_sc
  Constant2 : Constant  Value=AU
  Constant3 : Constant  Value=m
  Constant4 : Constant  Value=P
  Divide : Product  Inputs=*/  SaturateOnIntegerOverflow=on
  Divide1 : Product  Inputs=*/  SaturateOnIntegerOverflow=on
  Dot Product : DotProduct  OutDataTypeStr=Inherit: Inherit via internal rule
  Gain : Gain  Gain=-1  OutDataTypeStr=Inherit: Same as input  ParamDataTypeStr=Inherit: Same as input
  Normalize Vector : vrlib/Utilities/Normalize Vector  maxzero=0
  Product : Product  Inputs=6  SaturateOnIntegerOverflow=on
  Subtract : Sum  Inputs=+-
  a_srp : Outport
  wires:
  nu/1 -> Gain/1
  sun position/1 -> Subtract/1
  satellite position/1 -> Subtract/2
  Subtract/1 -> Normalize Vector/1, Dot Product/2, Dot Product/1
  Constant1/1 -> Product/1
  Constant/1 -> Product/2
  Gain/1 -> Product/3
  Normalize Vector/1 -> Product/4
  Dot Product/1 -> Divide/2
  Constant2/1 -> Divide/1
  Divide/1 -> Product/5
  Constant3/1 -> Divide1/2
  Product/1 -> Divide1/1
  Divide1/1 -> a_srp/1
  Constant4/1 -> Product/6

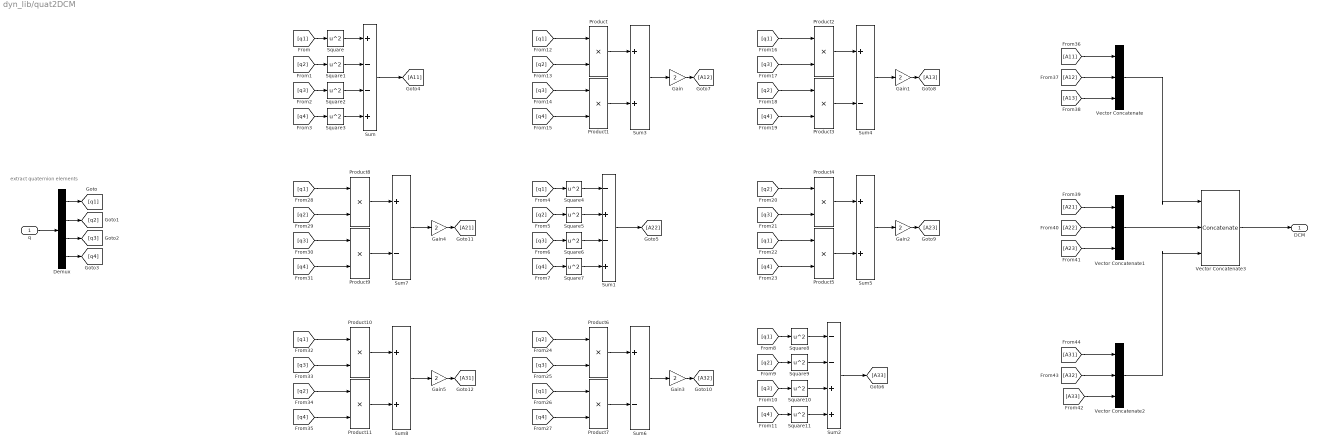
== system dyn_lib/quat2DCM ==
  note: extract quaternion elements
  q : Inport
  Demux : Demux
  Gain{,1..5} (6 alike) : Gain  Gain=2
  Product{,1..11} (12 alike) : Product
  Square{,1..11} (12 alike) : Math  Operator=square
  Sum : Sum  Inputs=+--+
  Sum1 : Sum  Inputs=-+-+
  Sum2 : Sum  Inputs=--++
  Sum3 : Sum
  Sum4 : Sum  Inputs=+-
  Sum5 : Sum
  Sum6 : Sum  Inputs=+-
  Sum7 : Sum  Inputs=+-
  Sum8 : Sum
  Vector Concatenate : Concatenate  NumInputs=3  Mode=Multidimensional array  ConcatenateDimension=2
  Vector Concatenate1 : Concatenate  NumInputs=3  Mode=Multidimensional array  ConcatenateDimension=2
  Vector Concatenate2 : Concatenate  NumInputs=3  Mode=Multidimensional array  ConcatenateDimension=2
  Vector Concatenate3 : Concatenate  NumInputs=3  Mode=Multidimensional array
  DCM : Outport
  wires:
  [q4] -> Product9/2
  [A33] -> Vector Concatenate2/3
  Vector Concatenate2/1 -> Vector Concatenate3/3
  [q2] -> Product8/2
  Square6/1 -> Sum1/3
  [A13] -> Vector Concatenate/3
  [q2] -> Product/2
  [q1] -> Product10/1
  [q1] -> Square4/1
  [A11] -> Vector Concatenate/1
  Square11/1 -> Sum2/4
  Vector Concatenate3/1 -> DCM/1
  [A31] -> Vector Concatenate2/1
  Vector Concatenate1/1 -> Vector Concatenate3/2
  Vector Concatenate/1 -> Vector Concatenate3/1
  [q2] -> Product6/1
  [q2] -> Product11/1
  Sum3/1 -> Gain/1
  [A32] -> Vector Concatenate2/2
  [q3] -> Product4/2
  [q1] -> Square8/1
  Demux/2 -> [q2]
  [A12] -> Vector Concatenate/2
  Gain3/1 -> [A32]
  Sum8/1 -> Gain5/1
  [q2] -> Product4/1
  [q3] -> Product9/1
  [A23] -> Vector Concatenate1/3
  [q3] -> Product6/2
  [A22] -> Vector Concatenate1/2
  [A21] -> Vector Concatenate1/1
  Square4/1 -> Sum1/1
  [q4] -> Product11/2
  Product8/1 -> Sum7/1
  Product4/1 -> Sum5/1
  Product10/1 -> Sum8/1
  Square8/1 -> Sum2/1
  [q3] -> Product10/2
  Product11/1 -> Sum8/2
  Square5/1 -> Sum1/2
  Product9/1 -> Sum7/2
  Sum7/1 -> Gain4/1
  [q4] -> Square11/1
  [q4] -> Product5/2
  Sum6/1 -> Gain3/1
  Sum5/1 -> Gain2/1
  [q4] -> Product7/2
  [q3] -> Square6/1
  Gain1/1 -> [A13]
  [q1] -> Product7/1
  Product3/1 -> Sum4/2
  Product7/1 -> Sum6/2
  [q1] -> Product5/1
  [q4] -> Product3/2
  [q3] -> Square2/1
  [q2] -> Square5/1
  [q3] -> Product1/1
  Product5/1 -> Sum5/2
  Product1/1 -> Sum3/2
  [q2] -> Square9/1
  [q3] -> Square10/1
  Square10/1 -> Sum2/3
  Sum4/1 -> Gain1/1
  Gain/1 -> [A12]
  Sum2/1 -> [A33]
  Product2/1 -> Sum4/1
  Square7/1 -> Sum1/4
  [q3] -> Product2/2
  Product/1 -> Sum3/1
  Square3/1 -> Sum/4
  [q1] -> Product/1
  Product6/1 -> Sum6/1
  [q2] -> Product3/1
  [q4] -> Product1/2
  Demux/3 -> [q3]
  Gain4/1 -> [A21]
  q/1 -> Demux/1
  [q1] -> Square/1
  Square2/1 -> Sum/3
  [q4] -> Square3/1
  Gain2/1 -> [A23]
  Demux/1 -> [q1]
  [q4] -> Square7/1
  Gain5/1 -> [A31]
  Sum1/1 -> [A22]
  Demux/4 -> [q4]
  [q1] -> Product2/1
  Sum/1 -> [A11]
  [q2] -> Square1/1
  Square9/1 -> Sum2/2
  Square1/1 -> Sum/2
  [q1] -> Product8/1
  Square/1 -> Sum/1

== system dyn_lib/shadow factor ==
  note: Computed the visible fraction of the sun disk given its apparend radius and occulted area
      |
      | Source:
      | O. Montenbruck and E. Gill, Satellite Orbits, Models, Methods and Applications
  note: Shadow factor
  Occulted Area : Inport
  Apparent sun radius : Inport  Port=2
  Constant : Constant
  Divide3 : Product  Inputs=*/
  Gain : Gain  Gain=pi  OutDataTypeStr=Inherit: Same as input  ParamDataTypeStr=Inherit: Same as input
  Min : MinMax  Inputs=2
  Square6 : Math  Operator=square
  Subtract2 : Sum  Inputs=+-
  shadow factor : Outport
  wires:
  Min/1 -> Divide3/1
  Subtract2/1 -> shadow factor/1
  Constant/1 -> Subtract2/1
  Gain/1 -> Divide3/2
  Apparent sun radius/1 -> Square6/1, Min/2
  Divide3/1 -> Subtract2/2
  Square6/1 -> Gain/1
  Occulted Area/1 -> Min/1

== system dyn_lib/Conical shadow/If Action Subsystem ==
  Action Port : ActionPort
  Constant : Constant  Value=0
  Occulted Area : Outport
  wires:
  Constant/1 -> Occulted Area/1

== system dyn_lib/Conical shadow/If Action Subsystem1 ==
  ar_sun : Inport
  Action Port : ActionPort
  Gain : Gain  Gain=pi  OutDataTypeStr=Inherit: Same as input  ParamDataTypeStr=Inherit: Same as input
  Square : Math  Operator=square
  Occulted area : Outport
  wires:
  ar_sun/1 -> Square/1
  Square/1 -> Gain/1
  Gain/1 -> Occulted area/1

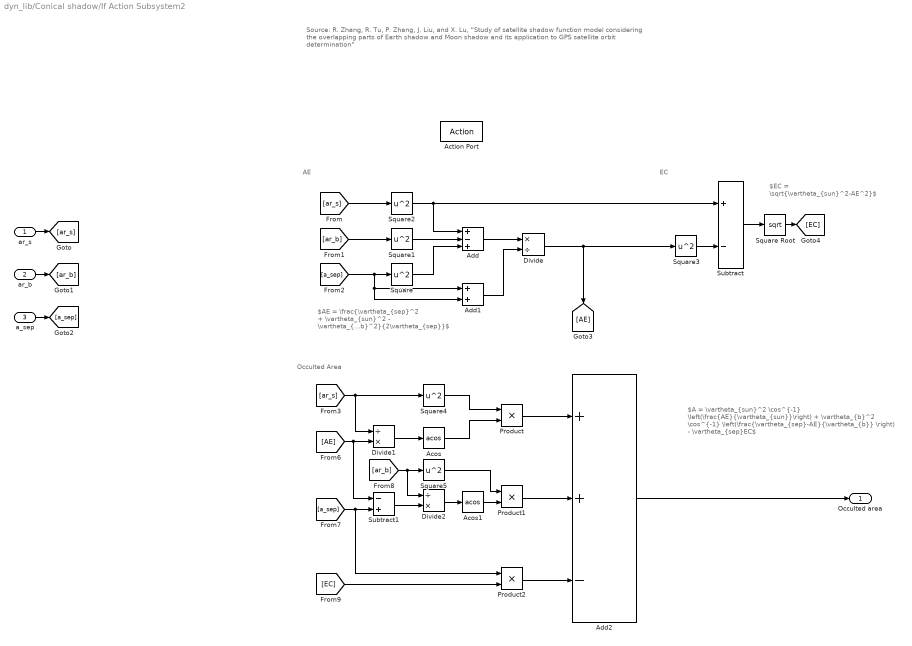
== system dyn_lib/Conical shadow/If Action Subsystem2 ==
  note: $A = \vartheta_{sun}^2 \cos^{-1} \left(\frac{AE}{\vartheta_{sun}}\right) + \vartheta_{b}^2 \cos^{-1} \left(\frac{\vartheta_{sep}-AE}{\vartheta_{b}} \right) - \vartheta_{sep}EC$
  note: $EC = \sqrt{\vartheta_{sun}^2-AE^2}$
  note: $AE = \frac{\vartheta_{sep}^2 + \vartheta_{sun}^2 - \vartheta_{b}^2}{2\vartheta_{sep}}$
  note: Source:
      | R. Zhang, R. Tu, P. Zhang, J. Liu, and X. Lu, “Study of satellite shadow function model considering the overlapping parts of Earth shadow and Moon shadow and its application to GPS satellite orbit determination”
  note: Occulted Area
  note: EC
  note: AE
  ar_s : Inport
  ar_b : Inport  Port=2
  a_sep : Inport  Port=3
  Action Port : ActionPort
  Acos : Trigonometry  Operator=acos
  Acos1 : Trigonometry  Operator=acos
  Add : Sum  Inputs=+-+
  Add1 : Sum
  Add2 : Sum  Inputs=++-
  Divide : Product  Inputs=*/
  Divide1 : Product  Inputs=/*
  Divide2 : Product  Inputs=/*
  Product : Product
  Product1 : Product
  Product2 : Product
  Square{,1..5} (6 alike) : Math  Operator=square
  Square Root : Sqrt
  Subtract : Sum  Inputs=+-
  Subtract1 : Sum  Inputs=-+
  Occulted area : Outport
  wires:
  ar_s/1 -> [ar_s]
  a_sep/1 -> [a_sep]
  ar_b/1 -> [ar_b]
  [a_sep] -> Add1/2, Add1/1, Square/1
  [ar_b] -> Square1/1
  [ar_s] -> Square2/1
  Square/1 -> Add/3
  Square1/1 -> Add/2
  Square2/1 -> Add/1, Subtract/1
  Add/1 -> Divide/1
  Add1/1 -> Divide/2
  Square3/1 -> Subtract/2
  Divide/1 -> Square3/1, [AE]
  Subtract/1 -> Square Root/1
  Square Root/1 -> [EC]
  [ar_s] -> Divide1/1, Square4/1
  [AE] -> Subtract1/1, Divide1/2
  Divide1/1 -> Acos/1
  Acos/1 -> Product/2
  Square4/1 -> Product/1
  [a_sep] -> Product2/1, Subtract1/2
  Subtract1/1 -> Divide2/2
  [ar_b] -> Square5/1, Divide2/1
  Divide2/1 -> Acos1/1
  Acos1/1 -> Product1/2
  Square5/1 -> Product1/1
  [EC] -> Product2/2
  Product2/1 -> Add2/3
  Product1/1 -> Add2/2
  Product/1 -> Add2/1
  Add2/1 -> Occulted area/1

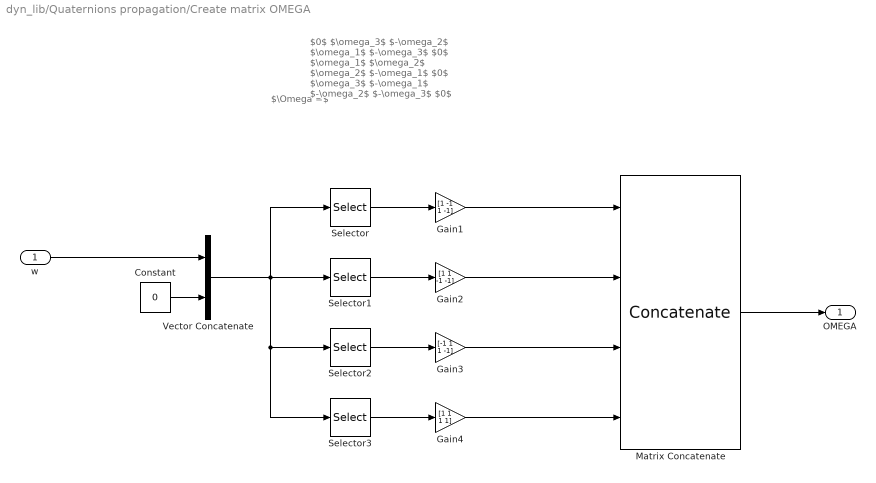
== system dyn_lib/Quaternions propagation/Create matrix OMEGA ==
  note: $\Omega =$
  note: $0$
      | $\omega_3$
      | $-\omega_2$
      | $\omega_1$
      |
      | $-\omega_3$
      | $0$
      | $\omega_1$
      | $\omega_2$
      |
      | $\omega_2$
      | $-\omega_1$
      | $0$
      | $\omega_3$
      |
      | $-\omega_1$
      | $-\omega_2$
      | $-\omega_3$
      | $0$
  w : Inport
  Constant : Constant  Value=0
  Gain1 : Gain  Gain=[1 -1 1 -1]
  Gain2 : Gain  Gain=[1 1 -1 -1]
  Gain3 : Gain  Gain=[-1 1 1 -1]
  Gain4 : Gain  Gain=[1 1 1 1]
  Matrix Concatenate : Concatenate  NumInputs=4  Mode=Multidimensional array  ConcatenateDimension=2
  Selector : Selector  InputPortWidth=4  IndexOptions=Index vector (dialog)  Indices=[4 3 2 1]  OutputSizes=1
  Selector1 : Selector  InputPortWidth=4  IndexOptions=Index vector (dialog)  Indices=[3 4 1 2]  OutputSizes=1
  Selector2 : Selector  InputPortWidth=4  IndexOptions=Index vector (dialog)  Indices=[2 1 4 3]  OutputSizes=1
  Selector3 : Selector  InputPortWidth=4  IndexOptions=Index vector (dialog)  Indices=[1 2 3 4]  OutputSizes=1
  Vector Concatenate : Concatenate
  OMEGA : Outport
  wires:
  Selector/1 -> Gain1/1
  Selector2/1 -> Gain3/1
  Selector3/1 -> Gain4/1
  Vector Concatenate/1 -> Selector/1, Selector1/1, Selector3/1, Selector2/1
  Constant/1 -> Vector Concatenate/2
  Selector1/1 -> Gain2/1
  Matrix Concatenate/1 -> OMEGA/1
  w/1 -> Vector Concatenate/1
  Gain1/1 -> Matrix Concatenate/1
  Gain2/1 -> Matrix Concatenate/2
  Gain3/1 -> Matrix Concatenate/3
  Gain4/1 -> Matrix Concatenate/4
